simulink model "lv_wind"  (Simulink 7.1)
settings: Solver=ode45  StartTime=0.0  StopTime=1000  RelTol=1e-3
settings Model: Creator=lv  LastModifiedBy=lv

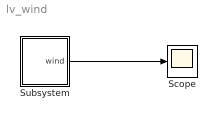
== system lv_wind ==
  Scope : Scope
      settings: SaveName=ScopeData9
  Subsystem : Subsystem
  wires:
  Subsystem/1(wind) -> Scope/1

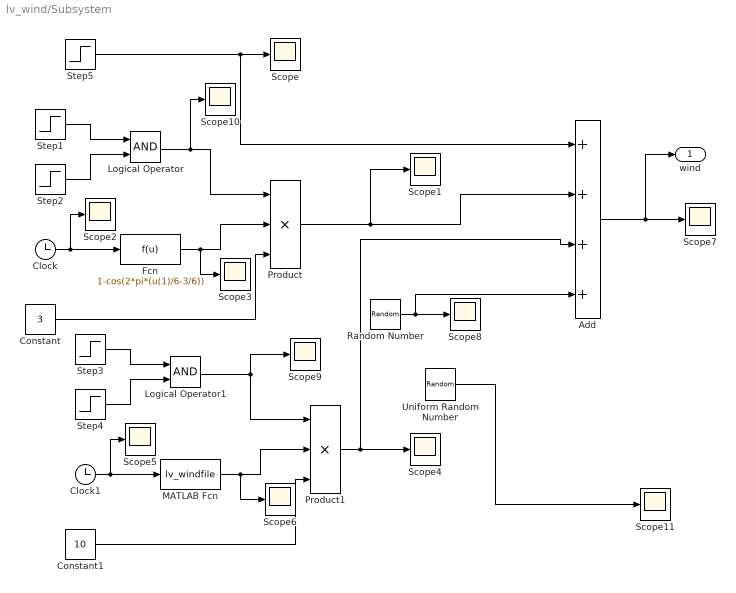
== system lv_wind/Subsystem ==
  Add : Sum  Inputs=++++  OutDataType=sfix(16)  OutScaling=2^-10
  Clock : Clock
  Clock1 : Clock
  Constant : Constant  Value=3  OutDataType=sfix(16)  OutScaling=2^0
  Constant1 : Constant  Value=10  OutDataType=sfix(16)  OutScaling=2^0
  Fcn : Fcn  Expr=1-cos(2*pi*(u(1)/6-3/6))
  Logical Operator : Logic  AllPortsSameDT=off  OutDataTypeMode=boolean  OutDataTypeStr=boolean
  Logical Operator1 : Logic  AllPortsSameDT=off  OutDataTypeMode=boolean  OutDataTypeStr=boolean
  MATLAB Fcn : MATLABFcn  MATLABFcn=lv_windfile
  Product : Product  Inputs=3  OutDataType=sfix(16)  OutScaling=2^0  RndMeth=Zero
  Product1 : Product  Inputs=3  OutDataType=sfix(16)  OutScaling=2^0  RndMeth=Zero
  Random Number : RandomNumber  SampleTime=0
  Scope{,1..11} (12 alike) : Scope
      Scope10 settings: SaveName=ScopeData11
      Scope11 settings: SaveName=ScopeData12
      Scope2 settings: SaveName=ScopeData2
      Scope3 settings: SaveName=ScopeData3
      Scope4 settings: SaveName=ScopeData4
      Scope5 settings: SaveName=ScopeData5
      Scope6 settings: SaveName=ScopeData6
      Scope7 settings: SaveName=ScopeData7
      Scope8 settings: SaveName=ScopeData8
      Scope9 settings: SaveName=ScopeData10
  Step1 : Step  Time=9  Before=1  After=0  SampleTime=0
  Step2 : Step  Time=3  SampleTime=0
  Step3 : Step  Time=11  Before=1  After=0  SampleTime=0
  Step4 : Step  Time=4  SampleTime=0
  Step5 : Step  Time=0  After=8  SampleTime=0
  Uniform Random Number : UniformRandomNumber  Minimum=3  Maximum=3.5  SampleTime=0
  wind : Outport  OutDataType=sfix(16)  OutScaling=2^0
  wires:
  Step5/1 -> Scope/1, Add/1
  Step1/1 -> Logical Operator/1
  Step2/1 -> Logical Operator/2
  Logical Operator/1 -> Product/1, Scope10/1
  Clock/1 -> Fcn/1, Scope2/1
  Fcn/1 -> Product/2, Scope3/1
  Constant/1 -> Product/3
  Product/1 -> Scope1/1, Add/2
  Step3/1 -> Logical Operator1/1
  Step4/1 -> Logical Operator1/2
  Logical Operator1/1 -> Product1/1, Scope9/1
  Clock1/1 -> Scope5/1, MATLAB Fcn/1
  MATLAB Fcn/1 -> Product1/2, Scope6/1
  Constant1/1 -> Product1/3
  Product1/1 -> Scope4/1, Add/3
  Add/1 -> Scope7/1, wind/1
  Random Number/1 -> Scope8/1, Add/4
  Uniform Random Number/1 -> Scope11/1
